simulink model "scdspeedtrigger"  (Simulink 6.0)
settings: Solver=ode45  StartTime=0.0  StopTime=60  MaxStep=0.01  RelTol=1e-3
model workspace (MAT data in the model file):
  p = [-7.82997288351e-05; 0.181210895977; -0.072497134344; 0.000486358314052; 0.0361674637937]
  xst.time = []
  xst.signals(1).values = 123.701650171
  xst.signals(1).dimensions = 1
  xst.signals(1).label = 'CSTATE'
  xst.signals(1).blockName = 'scdspeedtrigger/LTI System/Internal'
  xst.signals(2).values = 0.543634736226
  xst.signals(2).dimensions = 1
  xst.signals(2).label = 'CSTATE'
  xst.signals(2).blockName = 'scdspeedtrigger/Throttle & Manifold/Intake Manifold/p0 = 0.543 bar'
  xst.signals(3).values = 209.439510239
  xst.signals(3).dimensions = 1
  xst.signals(3).label = 'CSTATE'
  xst.signals(3).blockName = 'scdspeedtrigger/Vehicle
    | Dynamics/w = T//J
    | w0 = 209 rad//s'
  C.z = {-2.89}
  C.p = {0}
  C.k = 0.0018222
  C.Variable = 's'
  C.DisplayFormat = 'roots'
  C.lti.Ts = 0
  C.lti.ioDelay = 0
  C.lti.InputDelay = 0
  C.lti.OutputDelay = 0
  C.lti.InputName = {''}
  C.lti.OutputName = {''}
  C.lti.InputGroup = struct()
  C.lti.OutputGroup = struct()
  C.lti.Notes = {}
  C.lti.UserData = []
  C.lti.Version : numeric (value not decoded)
undefined symbols (not defined in the file or in its folder): sigbuilder_block
libraries: simulink x2, cstblocks x1, slctrlblks x1
settings Model: Creator=jglass  LastModifiedBy=jglass
settings DataIOCC: InitialState=[209.43951023932;123.701650171471;0.543634736225558]  LoadInitialState=on  SaveOutput=off  SaveTime=off
settings DebuggingCC: CheckExecutionContextPreStartOutputMsg=on  CheckExecutionContextRuntimeOutputMsg=on

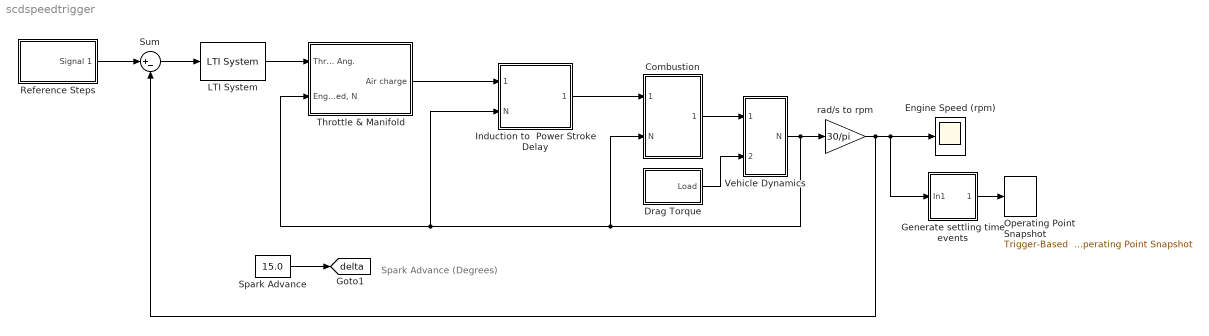
== system scdspeedtrigger ==
  note: Spark Advance
      | (Degrees)
  Combustion : Subsystem  PropExecContextAcrossSSBoundary=on
  Drag Torque : Subsystem  PropExecContextAcrossSSBoundary=on
  Engine Speed (rpm) : Scope
      settings: TickLabels=on  YMin=1500  YMax=3500  SaveName=N  DataFormat=Structure
  Generate settling time events : Subsystem  PropExecContextAcrossSSBoundary=on  mask(Settling Time Trigger Generator){ub=[2505;3005;3505], lb=[2495;2995;3495], interval=5}
      mask prompts: ub "Settling Time Upper Bounds"; lb "Settling Time Lower Bound"; interval "Settling Interval (sec.)"
      mask help: Generates trigger events for when a system comes to be within settling intervals specified in the block mask.
      mask init:
      | if length(ub) ~= length(lb)
      | 	error('The upper and lower bound settling time values must be the same.')
      | end
      mask Help:
      | <p>
      | The settling time trigger generator outputs trigger events for when a system comes to be within settling intervals specified in the block mask.
      | </p>
      | 
      | <p>
      | Mask variables:
      | </p>
      | <ul>
      | <li> Settling Time Upper Bounds - Upper limits for system settling.  This is a vector. </li>
      | <li> Settling Time Lower Bounds - Lower limits for system settling.  This is a vector. </li>
      | <li> Settling Interval - Time that a signal must be inside the settling region before a rising edge trigger is output from the block. </li>
      | </ul>
  Induction to  Power Stroke Delay : Subsystem  PropExecContextAcrossSSBoundary=on
  LTI System : cstblocks/LTI System  sys=C  IC=[]
  Operating Point Snapshot : slctrlblks/Trigger-Based  Operating Point Snapshot  Orientation=up  TriggerType=rising
  Reference Steps : Subsystem  Tag=STV Subsys  LoadFcn=sigbuilder_block('load');  StartFcn=sigbuilder_block('start');  StopFcn=sigbuilder_block('stop');  ClipboardFcn=sigbuilder_block('clipboard');  PropExecContextAcrossSSBoundary=on  mask(Sigbuilder block){}
      mask help: Sigbuilder GUI
      mask init:
      | if ~strcmp(get_param(bdroot(gcbh),'SimulationStatus'),'stopped') tuvar = sigbuilder_block('maskInit'); end
      settings: CopyFcn=sigbuilder_block('copy');  DeleteFcn=sigbuilder_block('delete');  ModelCloseFcn=sigbuilder_block('modelClose');  PreSaveFcn=sigbuilder_block('preSave');  NameChangeFcn=sigbuilder_block('namechange');  OpenFcn=sigbuilder_block('open',[50 50 520 400 ]);  CloseFcn=sigbuilder_block('close');
      mask Display: plot(0,0,100,100,[10,10,40,40,10],[80,20,20,80,80],[40,10],[50,50], [40,27,10],[65,72,56],[40,25,25,10],[28,28,43,43]);
  Spark Advance : Constant  Value=15.0
  Sum : Sum  Inputs=|+-
  Throttle & Manifold : Subsystem  PropExecContextAcrossSSBoundary=on
  Vehicle Dynamics : Subsystem  PropExecContextAcrossSSBoundary=on
  rad/s to rpm : Gain  Gain=30/pi  SaturateOnIntegerOverflow=on
  tag scope: delta=global
  wires:
  Throttle & Manifold/1(Air charge) -> Induction to  Power Stroke Delay/1(Air charge)
  Vehicle Dynamics/1(N) -> Combustion/2(N), Throttle & Manifold/2("Engine Speed, N"), Induction to  Power Stroke Delay/2(N), rad/s to rpm/1
  rad/s to rpm/1 -> Sum/2, Engine Speed (rpm)/1, Generate settling time events/1(In1)
  Combustion/1(Torque) -> Vehicle Dynamics/1(Teng)
  Drag Torque/1(Load) -> Vehicle Dynamics/2(Tload)
  Spark Advance/1 -> [delta]
  Induction to  Power Stroke Delay/1(Air Charge) -> Combustion/1(Air Charge)
  Reference Steps/1(Signal 1) -> Sum/1
  Sum/1 -> LTI System/1
  LTI System/1 -> Throttle & Manifold/1(Throttle Ang.)
  Generate settling time events/1(Out1) -> Operating Point Snapshot/Trigger

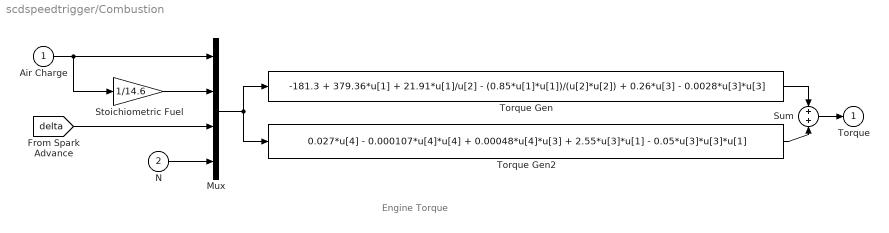
== system scdspeedtrigger/Combustion ==
  note: Engine Torque
  Air Charge : Inport  LatchInput=off
  N : Inport  Port=2  LatchInput=off
  Mux : Mux
  Stoichiometric Fuel : Gain  Gain=1/14.6  SaturateOnIntegerOverflow=on
  Sum : Sum  SaturateOnIntegerOverflow=on  InputSameDT=on
  Torque Gen : Fcn  Expr=-181.3 + 379.36*u[1] + 21.91*u[1]/u[2] - (0.85*u[1]*u[1])/(u[2]*u[2]) + 0.26*u[3] - 0.0028*u[3]*u[3]
  Torque Gen2 : Fcn  Expr=0.027*u[4] - 0.000107*u[4]*u[4] + 0.00048*u[4]*u[3] + 2.55*u[3]*u[1] - 0.05*u[3]*u[3]*u[1]
  Torque : Outport  InitialOutput=0
  wires:
  Stoichiometric Fuel/1 -> Mux/2
  [delta] -> Mux/3
  N/1 -> Mux/4
  Air Charge/1 -> Stoichiometric Fuel/1, Mux/1
  Mux/1 -> Torque Gen/1, Torque Gen2/1
  Torque Gen2/1 -> Sum/2
  Torque Gen/1 -> Sum/1
  Sum/1 -> Torque/1

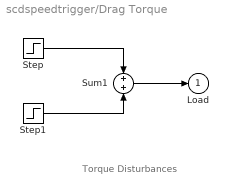
== system scdspeedtrigger/Drag Torque ==
  note: Torque Disturbances
  Step : Step  Time=2  Before=25  After=25  SampleTime=0
  Step1 : Step  Time=8  After=0  SampleTime=0
  Sum1 : Sum  SaturateOnIntegerOverflow=on  InputSameDT=on
  Load : Outport  InitialOutput=0
  wires:
  Step1/1 -> Sum1/2
  Step/1 -> Sum1/1
  Sum1/1 -> Load/1

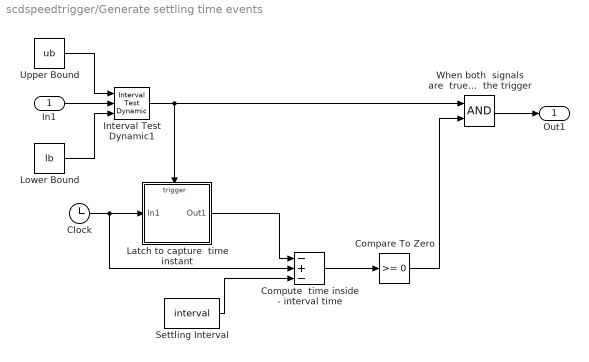
== system scdspeedtrigger/Generate settling time events ==
  In1 : Inport  LatchInput=off
  Clock : Clock
      settings: Decimation=10
  Compare To Zero : simulink/Logic and Bit Operations/Compare To Zero  relop=>=  LogicOutDataTypeMode=uint8
  "Compute  time inside - interval time  " : Sum  Inputs=-+-  OutDataTypeMode=double  OutScaling=2^-10
  Interval Test Dynamic1 : simulink/Logic and Bit Operations/Interval Test Dynamic  IntervalClosedRight=on  IntervalClosedLeft=on  LogicOutDataTypeMode=uint8
  Latch to capture  time instant : Subsystem  PropExecContextAcrossSSBoundary=on
  Lower Bound : Constant  Value=lb
  Settling Interval : Constant  Value=interval
  Upper Bound : Constant  Value=ub
  "When both  signals are  true throw  the trigger " : Logic  AllPortsSameDT=off  OutDataTypeMode=Boolean  LogicDataType=double
  Out1 : Outport
  wires:
  Settling Interval/1 -> "Compute  time inside - interval time  "/3
  "Compute  time inside - interval time  "/1 -> Compare To Zero/1
  Latch to capture  time instant/1(Out1) -> "Compute  time inside - interval time  "/1
  "When both  signals are  true throw  the trigger "/1 -> Out1/1
  Upper Bound/1 -> Interval Test Dynamic1/1
  In1/1 -> Interval Test Dynamic1/2
  Lower Bound/1 -> Interval Test Dynamic1/3
  Compare To Zero/1 -> "When both  signals are  true throw  the trigger "/2
  Clock/1 -> Latch to capture  time instant/1(In1), "Compute  time inside - interval time  "/2
  Interval Test Dynamic1/1 -> Latch to capture  time instant/Trigger, "When both  signals are  true throw  the trigger "/1

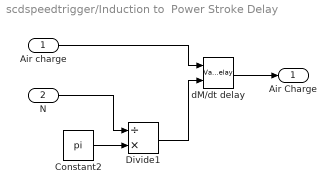
== system scdspeedtrigger/Induction to  Power Stroke Delay ==
  Air charge : Inport  LatchInput=off
  N : Inport  Port=2  LatchInput=off
  Constant2 : Constant  Value=pi
  Divide1 : Product  Inputs=/*  OutScaling=2^-10
  dM/dt delay : VariableTransportDelay  MaximumDelay=10  InitialInput=0.152  PadeOrder=2  TransDelayFeedthrough=on
  Air Charge : Outport
  wires:
  dM/dt delay/1 -> Air Charge/1
  Constant2/1 -> Divide1/2
  N/1 -> Divide1/1
  Divide1/1 -> dM/dt delay/2
  Air charge/1 -> dM/dt delay/1

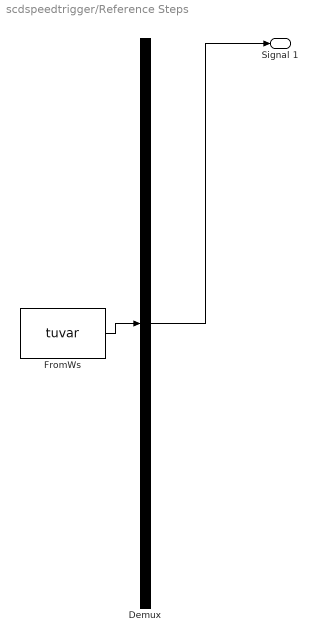
== system scdspeedtrigger/Reference Steps ==
  Demux : Demux  Tag=STV Demux  Outputs=1
  FromWs : FromWorkspace  Tag=STV FromWs  VariableName=tuvar  SampleTime=0  SigBuilderData=DataTag1  VnvData=DataTag2
      SigBuilderData=|
      | channels.label = 'Signal 1'
      | channels.allXData = {[0 2 2 20 20 40 40 60]}
      | channels.allYData = {[2000 2000 2500 2500 3000 3000 3500 3500]}
      | dataSet.timeRange = [0 60]
      | dataSet.name = 'Group 1'
  Signal 1 : Outport  Tag=STV Outport
  wires:
  Demux/1 -> Signal 1/1
  FromWs/1 -> Demux/1

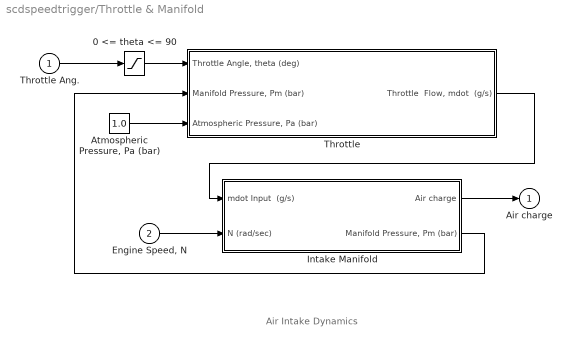
== system scdspeedtrigger/Throttle & Manifold ==
  note: Air Intake Dynamics
  Throttle Ang. : Inport  LatchInput=off
  "Engine Speed, N" : Inport  Port=2  LatchInput=off
  0 <= theta <= 90 : Saturate  UpperLimit=90  LowerLimit=0
  "Atmospheric Pressure, Pa (bar)" : Constant  Value=1.0
  Intake Manifold : Subsystem  PropExecContextAcrossSSBoundary=on
  Throttle : Subsystem  PropExecContextAcrossSSBoundary=on
  Air charge : Outport  InitialOutput=0
  wires:
  "Atmospheric Pressure, Pa (bar)"/1 -> Throttle/3("Atmospheric Pressure, Pa (bar) ")
  Intake Manifold/1(Air charge) -> Air charge/1
  Intake Manifold/2("Manifold Pressure, Pm (bar)") -> Throttle/2("Manifold Pressure, Pm (bar)")
  "Engine Speed, N"/1 -> Intake Manifold/2(N (rad/sec))
  Throttle/1("Throttle  Flow, mdot  (g/s)") -> Intake Manifold/1(mdot Input  (g/s))
  Throttle Ang./1 -> 0 <= theta <= 90/1
  0 <= theta <= 90/1 -> Throttle/1("Throttle Angle, theta (deg)")

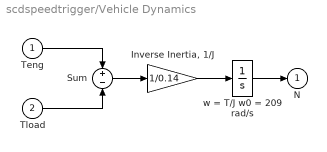
== system scdspeedtrigger/Vehicle Dynamics ==
  Teng : Inport  LatchInput=off
  Tload : Inport  Port=2  LatchInput=off
  "Inverse Inertia, 1/J" : Gain  Gain=1/0.14  SaturateOnIntegerOverflow=on
  Sum : Sum  Inputs=+-  SaturateOnIntegerOverflow=on  InputSameDT=on
  w = T/J w0 = 209 rad/s : Integrator  InitialCondition=209.48
  N : Outport  InitialOutput=0
  wires:
  "Inverse Inertia, 1/J"/1 -> w = T/J w0 = 209 rad/s/1
  w = T/J w0 = 209 rad/s/1 -> N/1
  Sum/1 -> "Inverse Inertia, 1/J"/1
  Teng/1 -> Sum/1
  Tload/1 -> Sum/2

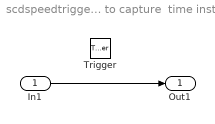
== system scdspeedtrigger/Generate settling time events/Latch to capture  time instant ==
  In1 : Inport  LatchInput=off
  Trigger : TriggerPort  OutputDataType=double  ZeroCross=off
  Out1 : Outport  InitialOutput=0
  wires:
  In1/1 -> Out1/1

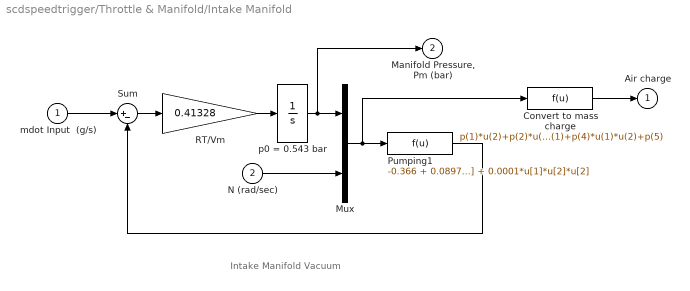
== system scdspeedtrigger/Throttle & Manifold/Intake Manifold ==
  note: Intake Manifold Vacuum
  mdot Input  (g/s) : Inport  LatchInput=off
  N (rad/sec) : Inport  Port=2  LatchInput=off
  Convert to mass charge : Fcn  Expr=p(1)*u(2)+p(2)*u(1)+p(3)*u(1)*u(1)+p(4)*u(1)*u(2)+p(5)
  Mux : Mux  Inputs=2
  Pumping1 : Fcn  Expr=-0.366 + 0.08979*u[1]*u[2] - 0.0337*u[2]*u[1]*u[1] + 0.0001*u[1]*u[2]*u[2]
  RT/Vm : Gain  Gain=0.41328  SaturateOnIntegerOverflow=on
  Sum : Sum  Inputs=|+-  SaturateOnIntegerOverflow=on  InputSameDT=on
  p0 = 0.543 bar : Integrator  InitialCondition=.543
  Air charge : Outport  InitialOutput=0
  "Manifold Pressure, Pm (bar)" : Outport  Port=2  InitialOutput=0
  wires:
  Pumping1/1 -> Sum/2
  Sum/1 -> RT/Vm/1
  p0 = 0.543 bar/1 -> "Manifold Pressure, Pm (bar)"/1, Mux/1
  Mux/1 -> Pumping1/1, Convert to mass charge/1
  N (rad/sec)/1 -> Mux/2
  RT/Vm/1 -> p0 = 0.543 bar/1
  mdot Input  (g/s)/1 -> Sum/1
  Convert to mass charge/1 -> Air charge/1

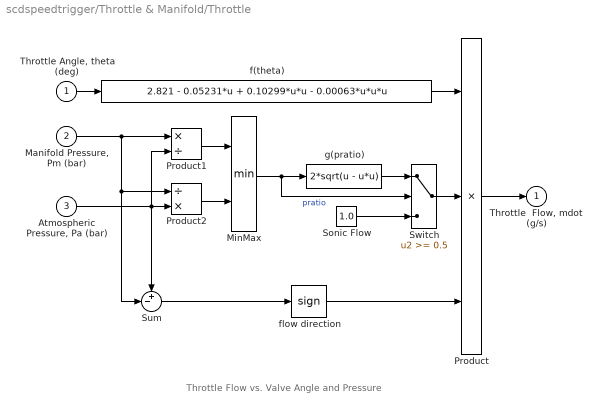
== system scdspeedtrigger/Throttle & Manifold/Throttle ==
  note: Throttle Flow vs. Valve Angle and Pressure
  "Throttle Angle, theta (deg)" : Inport  LatchInput=off
  "Manifold Pressure, Pm (bar)" : Inport  Port=2  LatchInput=off
  "Atmospheric Pressure, Pa (bar) " : Inport  Port=3  LatchInput=off
  MinMax : MinMax  Inputs=2  SaturateOnIntegerOverflow=on  InputSameDT=on
  Product : Product  Inputs=3  SaturateOnIntegerOverflow=on  RndMeth=Zero  InputSameDT=on
  Product1 : Product  Inputs=*/  SaturateOnIntegerOverflow=on  RndMeth=Zero  InputSameDT=on
  Product2 : Product  Inputs=/*  SaturateOnIntegerOverflow=on  RndMeth=Zero  InputSameDT=on
  "Sonic Flow " : Constant  Value=1.0
  Sum : Sum  Inputs=+-|  SaturateOnIntegerOverflow=on  InputSameDT=on
  Switch : Switch  Threshold=0.5  SaturateOnIntegerOverflow=on  InputSameDT=on
  f(theta) : Fcn  Expr=2.821 - 0.05231*u + 0.10299*u*u - 0.00063*u*u*u
  flow direction : Signum
  g(pratio) : Fcn  Expr=2*sqrt(u - u*u)
  "Throttle  Flow, mdot  (g/s)" : Outport  InitialOutput=0
  wires:
  f(theta)/1 -> Product/1
  Product/1 -> "Throttle  Flow, mdot  (g/s)"/1
  "Throttle Angle, theta (deg)"/1 -> f(theta)/1
  MinMax/1 -> g(pratio)/1, Switch/2  "pratio"
  Sum/1 -> flow direction/1
  flow direction/1 -> Product/3
  Switch/1 -> Product/2
  "Sonic Flow "/1 -> Switch/3
  g(pratio)/1 -> Switch/1
  "Atmospheric Pressure, Pa (bar) "/1 -> Product1/2, Product2/2, Sum/1
  Product1/1 -> MinMax/1
  Product2/1 -> MinMax/2
  "Manifold Pressure, Pm (bar)"/1 -> Product1/1, Product2/1, Sum/2
